simulink model "open_loop"  (R2017b)
settings: Solver=ode4  StartTime=0.0  StopTime=4  FixedStep=0.001  RelTol=1e-3
undefined symbols (not defined in the file): Kd, Ki, Km, Kp, Wm, Zm
settings Model: Creator=msi  LastModifiedBy=msi

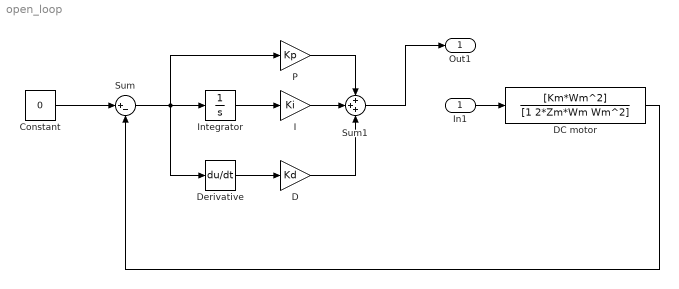
== system open_loop ==
  In1 : Inport
  Constant : Constant  Value=0
  D : Gain  Gain=Kd
  DC motor : TransferFcn  Numerator=[Km*Wm^2]  Denominator=[1 2*Zm*Wm Wm^2]
  Derivative : Derivative
  I : Gain  Gain=Ki
  Integrator : Integrator
  P : Gain  Gain=Kp
  Sum : Sum  Inputs=|+-
  Sum1 : Sum  Inputs=+++
  Out1 : Outport
  wires:
  Constant/1 -> Sum/1
  Sum/1 -> Derivative/1, P/1, Integrator/1
  Integrator/1 -> I/1
  Derivative/1 -> D/1
  P/1 -> Sum1/1
  I/1 -> Sum1/2
  D/1 -> Sum1/3
  DC motor/1 -> Sum/2
  Sum1/1 -> Out1/1
  In1/1 -> DC motor/1
